simulink model "Controller_sim"  (R2020b)
settings: Solver=VariableStepAuto  StartTime=0.0  StopTime=20  RelTol=1e-3
values from neighbouring files (symbols this model uses):
  F_mimo = -place(A,B,Desired_poles)    [SS_MIMO.m]
  J = [ -0.20692744238625918480350970935772, -0.23282465150808832388798617301067, -0.0018037394338624440108555852751087, -0.0027237770654514239686242003705982, -0.046616676828534540626855364172696, -0.0043748266894397930680961665394113 ... (first row only)    [SS_MIMO.m]    (also in SS_System.m; SS_ragnar_JS.m)
  L_mimo = -place(A',C',Desired_poles_obs)'    [SS_MIMO.m]
  M = M_tilde*N    [SS_MIMO.m]
  N = -(Ccl*Acl^-1*B_tilde_cl)^-1    [SS_MIMO.m]
  Ragnar_JS = ss(Ar,Br,Cr,0)    [SS_MIMO.m]    (also in SS_ragnar_JS.m)
  sys_k_mimo = ss(Ak_mimo,L_mimo,-F_mimo,0)    [SS_MIMO.m]
  sys_mimo = ss(A,B,C,0)    [SS_MIMO.m]
settings Model: Creator=krist  LastModifiedBy=krist

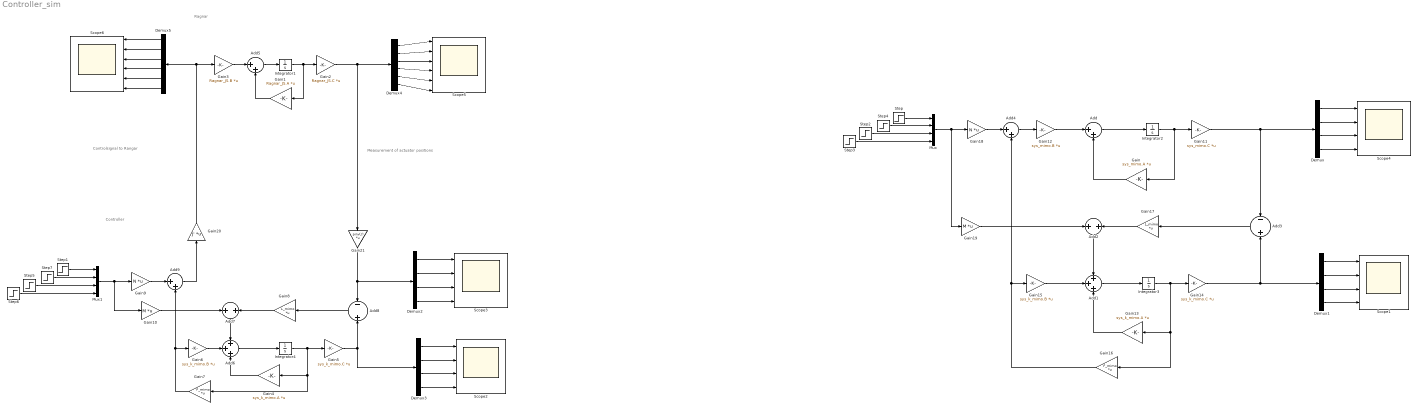
== system Controller_sim ==
  note: Ragnar
  note: Controller
  note: Measurement of
      | actuator positions
  note: Controlsignal
      | to Rangar
  Add{,4..5,9} (4 alike) : Sum  Inputs=|++
  Add1 : Sum  Inputs=+++
  Add2 : Sum
  Add3 : Sum  Inputs=-+
  Add6 : Sum  Inputs=+++
  Add7 : Sum
  Add8 : Sum  Inputs=-+
  Demux{,1..3} (4 alike) : Demux
  Demux4 : Demux  Outputs=6
  Demux5 : Demux  Outputs=6
  Gain : Gain  Gain=sys_mimo.A  Multiplication=Matrix(K*u)
  Gain1 : Gain  Gain=Ragnar_JS.A  Multiplication=Matrix(K*u)
  Gain10 : Gain  Gain=M  Multiplication=Matrix(K*u)
  Gain11 : Gain  Gain=sys_mimo.C  Multiplication=Matrix(K*u)
  Gain12 : Gain  Gain=sys_mimo.B  Multiplication=Matrix(K*u)
  Gain13 : Gain  Gain=sys_k_mimo.A  Multiplication=Matrix(K*u)
  Gain14 : Gain  Gain=sys_k_mimo.C  Multiplication=Matrix(K*u)
  Gain15 : Gain  Gain=sys_k_mimo.B  Multiplication=Matrix(K*u)
  Gain16 : Gain  Gain=F_mimo  Multiplication=Matrix(K*u)
  Gain17 : Gain  Gain=L_mimo  Multiplication=Matrix(K*u)
  Gain18 : Gain  Gain=N  Multiplication=Matrix(K*u)
  Gain19 : Gain  Gain=M  Multiplication=Matrix(K*u)
  Gain2 : Gain  Gain=Ragnar_JS.C  Multiplication=Matrix(K*u)
  Gain20 : Gain  Gain=J'  Multiplication=Matrix(K*u)
  Gain21 : Gain  Gain=pinv(J')  Multiplication=Matrix(K*u)
  Gain3 : Gain  Gain=Ragnar_JS.B  Multiplication=Matrix(K*u)
  Gain4 : Gain  Gain=sys_k_mimo.A  Multiplication=Matrix(K*u)
  Gain5 : Gain  Gain=sys_k_mimo.C  Multiplication=Matrix(K*u)
  Gain6 : Gain  Gain=sys_k_mimo.B  Multiplication=Matrix(K*u)
  Gain7 : Gain  Gain=F_mimo  Multiplication=Matrix(K*u)
  Gain8 : Gain  Gain=L_mimo  Multiplication=Matrix(K*u)
  Gain9 : Gain  Gain=N  Multiplication=Matrix(K*u)
  Integrator{1..4} (4 alike) : Integrator
  Mux : Mux
  Mux1 : Mux
  Scope{1..4} (4 alike) : Scope  NumInputPorts=4
  Scope5 : Scope  NumInputPorts=6
  Scope6 : Scope  NumInputPorts=6
  Step{,2..4} (4 alike) : Step  SampleTime=0
  Step1 : Step  Time=3  After=0  SampleTime=0
  Step5 : Step  Time=3  Before=-0.6  After=-0.4  SampleTime=0
  Step6 : Step  Time=3  After=deg2rad(90)  SampleTime=0
  Step7 : Step  Time=3  After=0.5  SampleTime=0
  wires:
  Demux/1 -> Scope4/1
  Step3/1 -> Mux/4
  Demux/4 -> Scope4/4
  Step/1 -> Mux/1
  Step2/1 -> Mux/3
  Demux/3 -> Scope4/3
  Gain12/1 -> Add/1
  Mux/1 -> Gain19/1, Gain18/1
  Add/1 -> Integrator2/1
  Integrator2/1 -> Gain/1, Gain11/1
  Demux/2 -> Scope4/2
  Gain/1 -> Add/2
  Gain11/1 -> Demux/1, Add3/1
  Step4/1 -> Mux/2
  Gain13/1 -> Add1/3
  Add1/1 -> Integrator3/1
  Integrator3/1 -> Gain16/1, Gain13/1, Gain14/1
  Gain15/1 -> Add1/2
  Gain14/1 -> Demux1/1, Add3/2
  Gain17/1 -> Add2/2
  Add2/1 -> Add1/1
  Gain18/1 -> Add4/1
  Add4/1 -> Gain12/1
  Gain19/1 -> Add2/1
  Gain16/1 -> Add4/2, Gain15/1
  Demux1/2 -> Scope1/2
  Demux1/3 -> Scope1/3
  Demux1/4 -> Scope1/4
  Demux1/1 -> Scope1/1
  Add3/1 -> Gain17/1
  Add8/1 -> Gain8/1
  Gain8/1 -> Add7/2
  Gain10/1 -> Add7/1
  Demux3/3 -> Scope2/3
  Demux3/4 -> Scope2/4
  Demux3/2 -> Scope2/2
  Gain5/1 -> Demux3/1, Add8/2
  Demux3/1 -> Scope2/1
  Step7/1 -> Mux1/2
  Demux2/2 -> Scope3/2
  Gain1/1 -> Add5/2
  Integrator1/1 -> Gain1/1, Gain2/1
  Add5/1 -> Integrator1/1
  Gain3/1 -> Add5/1
  Demux2/3 -> Scope3/3
  Step5/1 -> Mux1/3
  Demux2/4 -> Scope3/4
  Step6/1 -> Mux1/4
  Gain9/1 -> Add9/1
  Add6/1 -> Integrator4/1
  Step1/1 -> Mux1/1
  Gain4/1 -> Add6/3
  Add7/1 -> Add6/1
  Gain6/1 -> Add6/2
  Demux2/1 -> Scope3/1
  Integrator4/1 -> Gain7/1, Gain4/1, Gain5/1
  Gain20/1 -> Demux5/1, Gain3/1
  Gain21/1 -> Demux2/1, Add8/1
  Demux4/4 -> Scope5/4
  Demux4/3 -> Scope5/3
  Demux4/2 -> Scope5/2
  Demux4/1 -> Scope5/1
  Demux4/5 -> Scope5/5
  Demux4/6 -> Scope5/6
  Demux5/6 -> Scope6/6
  Demux5/4 -> Scope6/4
  Demux5/1 -> Scope6/1
  Demux5/2 -> Scope6/2
  Demux5/3 -> Scope6/3
  Demux5/5 -> Scope6/5
  Gain7/1 -> Gain6/1, Add9/2
  Mux1/1 -> Gain10/1, Gain9/1
  Add9/1 -> Gain20/1
  Gain2/1 -> Demux4/1, Gain21/1
